simulink library "rotationMatrices_ul"  (R2019a)
settings: Solver=VariableStepAuto  StartTime=0.0  StopTime=10.0  RelTol=1e-3
libraries: sharedutil x1
settings Model: Creator=jcreed2  LastModifiedBy=jcreed2

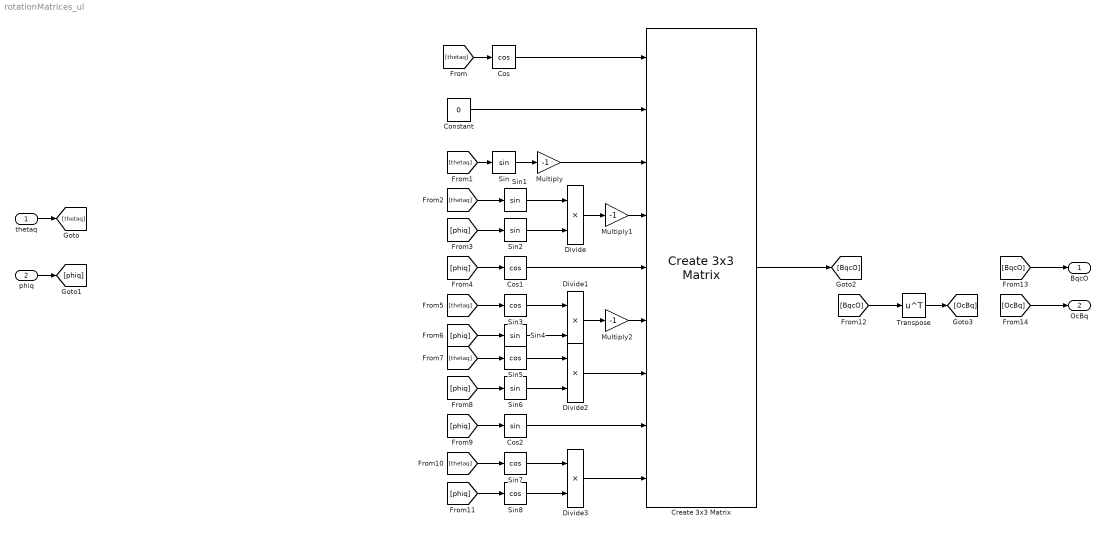
== system rotationMatrices_ul ==
  "thetaq " : Inport
  phiq : Inport  Port=2
  Constant : Constant  Value=0
  Cos : Trigonometry  Operator=cos
  Cos1 : Trigonometry  Operator=cos
  Cos2 : Trigonometry
  Create 3x3 Matrix : sharedutil/Create 3x3 Matrix  aMode=aMode
  Divide{,1..3} (4 alike) : Product  Inputs=**
  Multiply : Gain  Gain=-1
  Multiply1 : Gain  Gain=-1
  Multiply2 : Gain  Gain=-1
  Sin{,1..2,4,6} (5 alike) : Trigonometry
  Sin{3,5,7..8} (4 alike) : Trigonometry  Operator=cos
  Transpose : Math  Operator=transpose  SaturateOnIntegerOverflow=on
  BqcO : Outport
  OcBq : Outport  Port=2
  wires:
  Cos/1 -> Create 3x3 Matrix/1
  "thetaq "/1 -> [thetaq]
  phiq/1 -> [phiq]
  [thetaq] -> Cos/1
  Constant/1 -> Create 3x3 Matrix/2
  Multiply/1 -> Create 3x3 Matrix/3
  Sin/1 -> Multiply/1
  [thetaq] -> Sin/1
  Divide/1 -> Multiply1/1
  Sin1/1 -> Divide/1
  Sin2/1 -> Divide/2
  [thetaq] -> Sin1/1
  [phiq] -> Sin2/1
  Multiply1/1 -> Create 3x3 Matrix/4
  Cos1/1 -> Create 3x3 Matrix/5
  [phiq] -> Cos1/1
  Divide1/1 -> Multiply2/1
  Sin4/1 -> Divide1/2
  Sin3/1 -> Divide1/1
  [phiq] -> Sin4/1
  [thetaq] -> Sin3/1
  Multiply2/1 -> Create 3x3 Matrix/6
  [phiq] -> Sin6/1
  Sin6/1 -> Divide2/2
  Sin5/1 -> Divide2/1
  [thetaq] -> Sin5/1
  Divide2/1 -> Create 3x3 Matrix/7
  [phiq] -> Cos2/1
  Cos2/1 -> Create 3x3 Matrix/8
  Sin8/1 -> Divide3/2
  [thetaq] -> Sin7/1
  Sin7/1 -> Divide3/1
  [phiq] -> Sin8/1
  Divide3/1 -> Create 3x3 Matrix/9
  Create 3x3 Matrix/1 -> [BqcO]
  [BqcO] -> Transpose/1
  Transpose/1 -> [OcBq]
  [BqcO] -> BqcO/1
  [OcBq] -> OcBq/1
